simulink model "ava5"  (R2017b)
settings: Solver=VariableStepAuto  StartTime=0.0  StopTime=10.0  RelTol=1e-3
settings Model: Creator=hbourbou  LastModifiedBy=hbourbou

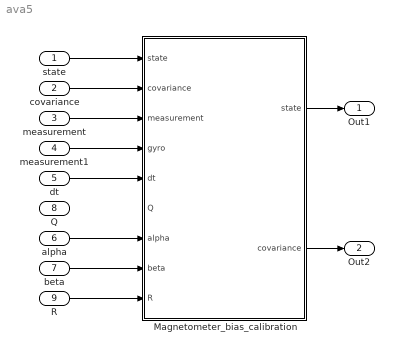
== system ava5 ==
  state : Inport  PortDimensions=6
  covariance : Inport  Port=2  PortDimensions=[6, 6]
  measurement : Inport  Port=3  PortDimensions=3
  measurement1 : Inport  Port=4  PortDimensions=3
  dt : Inport  Port=5
  alpha : Inport  Port=6
  beta : Inport  Port=7
  Q : Inport  Port=8  PortDimensions=[6, 6]
  R : Inport  Port=9  PortDimensions=[3, 3]
  Magnetometer_bias_calibration : MATLAB Function  TreatAsAtomicUnit=on
  Out1 : Outport
  Out2 : Outport  Port=2
  wires:
  state/1 -> Magnetometer_bias_calibration/1("state ")
  covariance/1 -> Magnetometer_bias_calibration/2("covariance ")
  measurement/1 -> Magnetometer_bias_calibration/3(measurement)
  measurement1/1 -> Magnetometer_bias_calibration/4(gyro)
  dt/1 -> Magnetometer_bias_calibration/5(dt)
  alpha/1 -> Magnetometer_bias_calibration/7(alpha)
  beta/1 -> Magnetometer_bias_calibration/8(beta)
  R/1 -> Magnetometer_bias_calibration/9(R)
  Magnetometer_bias_calibration/1(state) -> Out1/1
  Magnetometer_bias_calibration/2(covariance) -> Out2/1

== matlab function ava5/Magnetometer_bias_calibration ==
  data: state input; state output; covariance input; measurement input; gyro input; dt input; Q input; alpha input; beta input; R input; covariance output
function [state, covariance]=filter_byAngularVelocity(state,covariance,measurement, gyro,dt,Q,alpha,beta,R)
    
z=measurement;
w=gyro;
UKFx=state; UKFP=covariance;
[X,W] = computeSigmaPoints(UKFx,UKFP);

% Propagate sigma points through transition function
Xkk1 = X;
for i=1:size(X,2)
    Xkk1(1:size(UKFx,1),i) = X(:,i)+ dt*[-skew(w) skew(w);zeros(3,3) zeros(3,3)]* X(:,i);
end

% Recombine weighted sigma points to produce predicted state and covariance
xkk1 = Xkk1*W;%wmean(Xkk1,W);      
Pkk1 = wcov(Xkk1,W,alpha,beta) + Q;

% propagate sigma points through observation function
Zkk1=Xkk1(1:3,:); %measurement = state

% Recombine weighted sigma points to produce predicted measurement and covariance
zkk1 =Zkk1*W;% wmean(Zkk1,W);
Pzz =  wcov(Zkk1,W,alpha,beta) + R;

% 2. Update
% Compute state-measurement cross-covariance matrix
Pxz = zeros(6,3);
for i=1:length(W)
    Pxz = Pxz + W(i)*(Xkk1(:,i)-xkk1)*(Zkk1(:,i)-zkk1)';
end
Pxz = Pxz + (1-alpha^2+beta)*(Xkk1(:,1)-xkk1)*(Zkk1(:,1)-zkk1)';
Kk = Pxz/Pzz;% Compute kalman gain

xk1 = xkk1 + Kk*(z-zkk1);% Compute state and measurement estimates
Pk1 = Pkk1 - Kk*Pzz*Kk';

covariance=Pk1;
state =xk1;
%calibrated_measurement=xk1(1:3)-xk1(4:6);
end

function [X,W,mX,PX] = computeSigmaPoints(mx,Pxx)
% computeSigmaPoints   Sigma point calculation
%   computes a set of sigma points defined by samples X and weights W,
%   given mean mx, covariance Pxx, a sigma point method, free parameters, a
%   scaling parameter, and a matrix square root function.
%%   X will be formatted such that the rows are variables and the columns
%   are samples. W will be a row vector. mx must be a column vector. Pxx
%   must be a square matrix.

alpha = 1; % Set default options
n = size(mx,1);% Compute number of samples
beta=2;% Check for beta parameter
kappa = 0;% Compute sigma points

X=zeros(6,2*n+1);
X(1:6,1) = mx;% Compute unscaled sigma points
matrixSq = Cholp((n+kappa)*Pxx)';
X(1:6,2:n+1) = repmat(mx,1,n) + matrixSq;
X(1:6,n+2:2*n+1) = repmat(mx,1,n) - matrixSq;


W=zeros(2*n+1,1);% Compute weights
W(1) = kappa/(n+kappa); W(2:2*n+1) = .5/(n+kappa);

p = size(X,2);% Scale the sigma points
X = repmat(X(:,1),1,p) + alpha*(X-repmat(X(:,1),1,p));

W(1) = W(1)/alpha^2 + (1-1/alpha^2);W(2:end) = W(2:end)/alpha^2;% Compute weights


mX = X*W; %wmean(X,W);% Compute weighted mean and covariance
PX = wcov(X,W,alpha,beta);


end


function Pxx = wcov(X,w,alpha,beta)
% wcov   Weighted covariance calculation
mX = X*w;% wmean(X,w);%weighted mean

Pxx =zeros(size(X,1),size(X,1));
for i=1:size(X,2)
    Pxx = Pxx + w(i)*(X(:,i)-mX)*(X(:,i)-mX)';
end
Pxx = Pxx + (1-alpha^2+beta)*(X(:,1)-mX)*(X(:,1)-mX)';
end

function R=Cholp(A)
   % CHOLESKY computes the Cholesky decomposition of a matrix
   %   R=Cholesky(A) computes the Cholesky decomposition A=R'R
   R=zeros(size(A,1));
   n=length(A);
   for j=1:n
       v=A(j,j:n);
       if j>1
           v=A(j,j:n)-R(1:j-1,j)'*R(1:j-1,j:n);
       end 
       if v(1)<=0
           R=eye(size(A,1));%error('Matrix is not positive definite')
           return;
       else
           h=1/sqrt(v(1));
       end
       R(j,j:n)=v*h;
   end
end

function xhat = skew(x)
% Computes the hat map, mapping a 3-vector into a 3X3 skew-symmetric matrix
xhat = [  0   -x(3)  x(2)
    x(3)   0   -x(1)
    -x(2)  x(1)  0];

end

% function mX = wmean(X,w)
% % wmean   Weighted mean calculation
% %
% %   mX = wmean(X,w) computes the weighted mean given samples X and weights
% %   w.
% %
% %   X must be formatted such that the rows are variables and the columns
% %   are samples. If X is a vector, then both X and w can be either row or
% %   column vectors.%
% 
% % Ensure that if X is a vector, then both X and w are column vectors
% if size(X,2)==1
%     % Then X is a column vector, make it a row vector (for the
%     % multiplication)
%     X = X';
% end
% if size(w,1)==1
%     % Then w is a row vector, make it a column vector
%     w = w';
% end
% 
% % Compute weighted mean
% mX = X*w;
% end
